simulink model "demodOOK_done"  (R2018a)
settings: Solver=VariableStepAuto  StartTime=0.0  StopTime=10.0  RelTol=1e-3
model workspace (MAT data in the model file):
  Sig = Simulink.Signal
  Sig.DataType = 'auto'
  Sig.Dimensions = -1
  Sig.DimensionsMode = 'auto'
  Sig.Complexity = 'auto'
  Sig.SampleTime = -1
  Sig.SamplingMode = 'auto'
  l = 39
  logsout = Simulink.SimulationData.Dataset
  logsout.any.Name = 'logsout'
  logsout.any.Version = 3
  logsout.any.Storage = Simulink.SimulationData.Storage.RamDatasetStorage
  logsout.any.Storage.any.Version = 2
  logsout.any.Storage.any.Elements{1} = Simulink.SimulationData.Signal
  logsout.any.Storage.any.Elements{1}.PortType = 'outport'
  logsout.any.Storage.any.Elements{1}.Version = 1
  logsout.any.Storage.any.Elements{1}.BlockPath = Simulink.SimulationData.BlockPath
  logsout.any.Storage.any.Elements{1}.BlockPath.path = {'demodOOK/Remove Preamble'}
  logsout.any.Storage.any.Elements{1}.Values = timeseries
  logsout.any.Storage.any.Elements{1}.Values.DataInfo = tsdata.datametadata
  logsout.any.Storage.any.Elements{1}.Values.DataInfo.Interpolation = tsdata.interpolation
  logsout.any.Storage.any.Elements{1}.Values.DataInfo.Interpolation.Fhandle : function handle (value not decoded)
  logsout.any.Storage.any.Elements{1}.Values.DataInfo.Interpolation.Name = 'zoh'
  logsout.any.Storage.any.Elements{1}.Values.TimeInfo = tsdata.timemetadata
  logsout.any.Storage.any.Elements{1}.Values.TimeInfo.Length = 74
  logsout.any.Storage.any.Elements{1}.Values.TimeInfo.DuplicateTimes = 0
  logsout.any.Storage.any.Elements{1}.Values.TimeInfo.Increment_ = 0.136
  logsout.any.Storage.any.Elements{1}.Values.TimeInfo.Start_ = 0
  logsout.any.Storage.any.Elements{1}.Values.TimeInfo.Initialized = 1
  logsout.any.Storage.any.Elements{1}.Values.QualityInfo = tsdata.qualmetadata
  logsout.any.Storage.any.Elements{1}.Values.Data_ = [0 0 0 0 0 0 0 0 0 0 0 0 ... (27232 elements, 368x1x74)]
  logsout.any.Storage.any.Elements{1}.Values.IsTimeFirst_ = 0
  rec.msg_len = 46
  rec.ascii_len = 8
  rec.fs = 3000
  rec.preamble = [1 1 1 1 1 1 1 1 1 1 1 1 1 1 1 0 0 0 0 0 0 1 1 1 1 1 1 0 0 0 1 1 1 0 0 0 1 1 1]
  rec.preamble_len = 39
  rec.preamble_pad_len = 1
  rec.preamble_pad = 0
  rec.frame_pad_len = 2
  rec.frame_pad = [0 0]
  rec.master_msg_len = 368
  rec.master_frame_len = 410
  rec.filter_coeff = [1 1 1 -1 -1 -1 1 1 1 -1 -1 -1 1 1 1 1 1 1 -1 -1 -1 -1 -1 -1 1 1 1 1 1 1 1 1 1 1 1 1 1 1 1]
  rec.filter_coeff_odd = [1 1 -1 1 1 -1 1 1 1 -1 -1 -1 1 1 1 1 1 1 1 1]
  rec.filter_coeff_even = [1 -1 -1 1 -1 -1 1 1 1 -1 -1 -1 1 1 1 1 1 1 1]
  tout = [0 2.08333333333e-05 4.16666666667e-05 6.25e-05 8.33333333333e-05 0.000104166666667 0.000125 0.000145833333333 0.000166666666667 0.0001875 0.000208333333333 0.000229166666667 ... (480001 elements, 480001x1)]
libraries: simulink x3, commutil2 x2, simulink_need_slupdate x2, dspfdesign x2, dspsnks4 x1, rtlsdr_book_library x1, dspvision x1, dspstat3 x1, dspmtrx3 x1
(part 1 of 2)
settings Model: Creator=krist  LastModifiedBy=krist

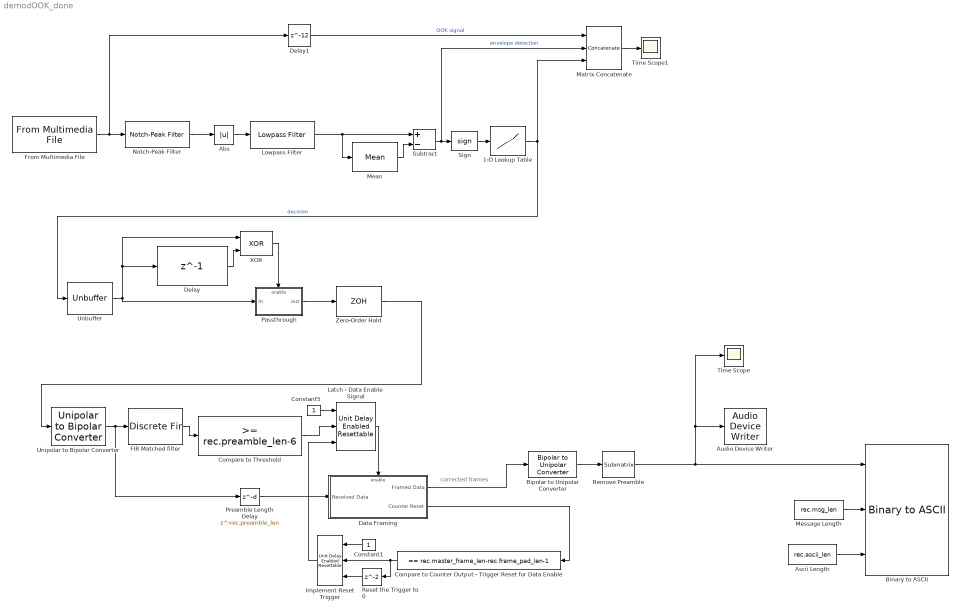
== system demodOOK_done ==
  note: corrected frames
  1-D Lookup Table : Lookup_n-D  NumberOfTableDimensions=1  BreakpointsForDimension1=[-1,0,1]  Table=[0,0,1]  InternalRulePriority=Speed  RndMeth=Simplest  InputSameDT=on
  Abs : Abs
  Ascii Length : Constant  Value=rec.ascii_len  VectorParams1D=off  OutDataTypeStr=single  FramePeriod=4096/240e3
  Audio Device Writer : dspsnks4/Audio Device Writer  Driver=DirectSound  Device=Default  InheritSampleRate=on  SampleRate=44100  BitDepth=16-bit integer  BufferSize=4096  NumBuffers=10  DefaultOutputChannelMapping=on  OutputChannelMapping=1:2  OutputNumUnderrunSamples=off  DriverIdx=1  DeviceWarnFlag=''
  Binary to ASCII : rtlsdr_book_library/Data Comms Sources and Sinks/ASCII Decoding/Binary to ASCII  SystemSampleTime=-1
      settings: SourceProductName=RTL-SDR Book Library
  Bipolar to Unipolar Converter : commutil2/Bipolar to Unipolar Converter  M=2  polarity=Positive  dataType=Inherit via internal rule
      settings: SourceProductName=Communications System Toolbox  SourceProductBaseCode=CM
  Compare to Counter Output - Trigger Reset for Data Enable : simulink/Logic and Bit Operations/Compare To Constant  relop===  const=rec.master_frame_len-rec.frame_pad_len-1  OutDataTypeStr=boolean
  Compare to Threshold : simulink/Logic and Bit Operations/Compare To Constant  relop=>=  const=rec.preamble_len-6  OutDataTypeStr=boolean
  Constant1 : Constant
  Constant5 : Constant
  Data Framing : Subsystem
  Delay : Delay  DelayLength=1  InitialCondition=0
  Delay1 : Delay  DelayLength=12  InputProcessing=Columns as channels (frame based)
  FIR Matched filter : DiscreteFir  Coefficients=rec.filter_coeff  InputProcessing=Columns as channels (frame based)
  From Multimedia File : dspvision/From Multimedia File  inputFilename=C:\Users\krist\Documents\gitstuff\tg19hack\misc\So music\src\testmix.ogg  loop=on  numPlays=inf  outputStreams=Audio only  videoDataType=single  audioDataType=double  inheritSampleTime=on  userDefinedSampleTime=1/30  noAudioOutput=off  isIntensityVideo=off  fourcc=RGB  colorVideoFormat=Separate color signals  outputEOF=off  dataOrg=Column-major  audioFrameSize=1024  computeAudioFrameSize=off  outSamplingMode=Sample based
      settings: SourceProductBaseCode=VP
  Implement Reset Trigger : simulink_need_slupdate/Unit Delay Enabled Resettable  vinit=0  tsamp=-1
      settings: SourceProductName=Simulink  SourceProductBaseCode=SL
  Latch - Data Enable Signal : simulink_need_slupdate/Unit Delay Enabled Resettable  vinit=0  tsamp=-1
      settings: SourceProductName=Simulink  SourceProductBaseCode=SL
  Lowpass Filter : dspfdesign/Lowpass Filter  FilterType=FIR  DesignForMinimumOrder=off  FilterOrder=20  PassbandFrequency=1.5e3  StopbandFrequency=3e3  PassbandRipple=0.1  StopbandAttenuation=80  InheritSampleRate=off  SampleRate=48e3  SimulateUsing=Interpreted execution  roundingMode=Floor  coeffsDataTypeStr=fixdt(1,16)
  Matrix Concatenate : Concatenate  NumInputs=3  Mode=Multidimensional array  ConcatenateDimension=2
  Mean : dspstat3/Mean  run=off  InputProcessing=Columns as channels (frame based)  reset_popup=None  directionMode=Each column  dimension=1  roiEnable=off  roiType=Rectangles  roiPortion=Entire ROI  roiOutput=Individual statistics for each ROI  roiFlag=off  roundingMode=Floor  overflowMode=off  outputDataTypeStr=Inherit: Same as accumulator  outputMin=[]  outputMax=[]  outputLastDataTypeStr=Inherit: Same as accumulator
  Message Length : Constant  Value=rec.msg_len  VectorParams1D=off  OutDataTypeStr=single  FramePeriod=-1
  Notch-Peak Filter : dspfdesign/Notch-Peak Filter  Specification=Bandwidth and center frequency  BandwidthPort=off  Bandwidth=2205  QualityFactorPort=off  QualityFactor=5  CenterFrequencyPort=off  CenterFrequency=12000  BandwidthCoefficientPort=off  BandwidthCoefficient=0.72654  CenterFrequencyCoefficientPort=off  CenterFrequencyCoefficient=0  Output=Peak  InheritSampleRate=off  SampleRate=48000  SimulateUsing=Interpreted execution
      settings: SourceProductName=DSP System Toolbox  SourceProductBaseCode=DS
  Passthrough : Subsystem
  Preamble Length Delay : Delay  DelayLength=rec.preamble_len  DelayLengthUpperLimit=10000  InitialCondition=1
  Remove Preamble : dspmtrx3/Submatrix  RowSpan=Range of rows  RowStartMode=Index  RowStartIndex=rec.preamble_len+rec.preamble_pad_len+1  RowEndMode=Index  RowEndIndex=rec.master_frame_len-rec.frame_pad_len  ColSpan=One column  ColStartMode=First  ColStartIndex=1  ColEndMode=Last  ColEndIndex=1
  Reset the Trigger to 0 : Delay  DelayLengthUpperLimit=10000  InitialCondition=0
  Sign : Signum  ZeroCross=off
  Subtract : Sum  Inputs=+-
  Time Scope : Scope
  Time Scope1 : Scope
      settings: StartFcn=startfcn_time_scope
  Unbuffer : Unbuffer
  Unipolar to Bipolar Converter : commutil2/Unipolar to Bipolar Converter  M=2  polarity=Positive  dataType=Inherit via internal rule
      settings: SourceProductName=Communications System Toolbox
  XOR : Logic  Operator=XOR  IconShape=distinctive  AllPortsSameDT=off  OutDataTypeStr=boolean
  Zero-Order Hold : ZeroOrderHold  SampleTime=1/3e3
  wires:
  Notch-Peak Filter/1 -> Abs/1
  Abs/1 -> Lowpass Filter/1
  Lowpass Filter/1 -> Mean/1, Subtract/1
  Mean/1 -> Subtract/2
  Sign/1 -> 1-D Lookup Table/1
  From Multimedia File/1 -> Delay1/1, Notch-Peak Filter/1
  Matrix Concatenate/1 -> Time Scope1/1
  Delay1/1 -> Matrix Concatenate/1  "OOK signal"
  Subtract/1 -> Matrix Concatenate/2, Sign/1  "envelope detection"
  1-D Lookup Table/1 -> Unbuffer/1, Matrix Concatenate/3  "decision"
  Delay/1 -> XOR/2
  Unbuffer/1 -> XOR/1, Delay/1, Passthrough/1(in)
  XOR/1 -> Passthrough/Enable
  Passthrough/1(out) -> Zero-Order Hold/1
  Data Framing/1(Framed Data) -> Bipolar to Unipolar Converter/1
  Latch - Data Enable Signal/1 -> Data Framing/Enable
  FIR Matched filter/1 -> Compare to Threshold/1
  Compare to Threshold/1 -> Latch - Data Enable Signal/2
  Implement Reset Trigger/1 -> Latch - Data Enable Signal/3
  Zero-Order Hold/1 -> Unipolar to Bipolar Converter/1
  Constant1/1 -> Implement Reset Trigger/1
  Constant5/1 -> Latch - Data Enable Signal/1
  Compare to Counter Output - Trigger Reset for Data Enable/1 -> Implement Reset Trigger/2, Reset the Trigger to 0/1
  Data Framing/2(Counter Reset) -> Compare to Counter Output - Trigger Reset for Data Enable/1
  Unipolar to Bipolar Converter/1 -> FIR Matched filter/1, Preamble Length Delay/1
  Bipolar to Unipolar Converter/1 -> Remove Preamble/1
  Preamble Length Delay/1 -> Data Framing/1(Received Data)
  Reset the Trigger to 0/1 -> Implement Reset Trigger/3
  Message Length/1 -> Binary to ASCII/2
  Ascii Length/1 -> Binary to ASCII/3
  Remove Preamble/1 -> Time Scope/1, Audio Device Writer/1, Binary to ASCII/1
